simulink model "UAV"  (R2018a)
settings: Solver=VariableStepAuto  StartTime=0.0  StopTime=10.0  RelTol=1e-3
values from neighbouring files (symbols this model uses):
  A = [0 0 1 0 0 0 0.0009 0 0 ... (first row only)    [model.m]    (also in model_disturbance.m)
  B = [0 0 0 ... (first row only)    [model.m]    (also in model_disturbance.m)
  C = [1 0 0 0 0 0 0 0 0 ... (first row only)    [model.m]    (also in model_disturbance.m)
  D = zeros(6,3)    [model.m]    (also in model_disturbance.m = zeros(6,6))
  M = A-B*K-l*C    [model.m]    (also in model_disturbance.m)
undefined symbols (not defined in the file or in its folder): K, l
settings Model: Creator=HP  LastModifiedBy=HP

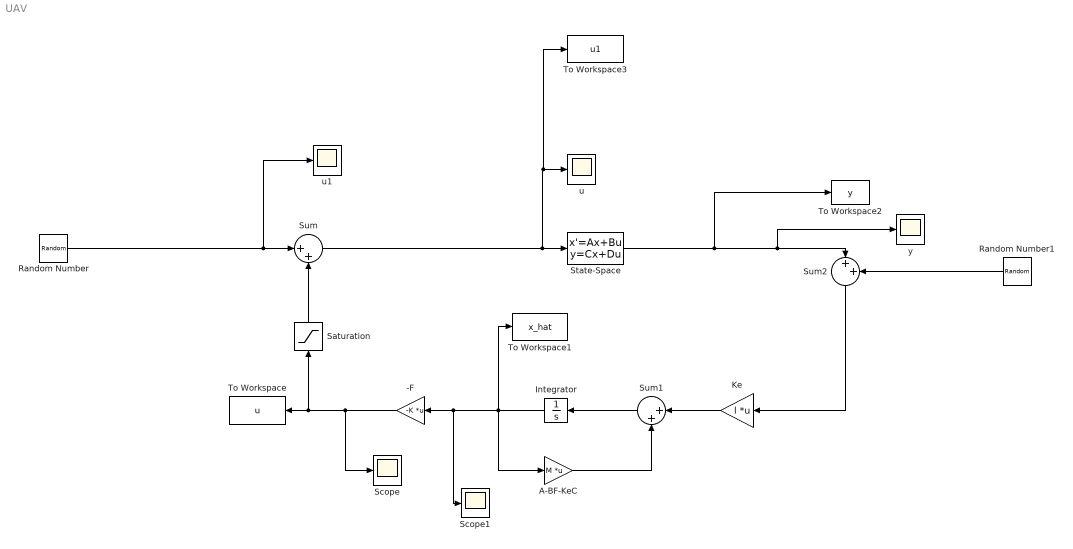
== system UAV ==
  " -F" : Gain  Gain=-K  Multiplication=Matrix(K*u) (u vector)
  A-BF-KeC : Gain  Gain=M  Multiplication=Matrix(K*u) (u vector)
  Integrator : Integrator  InitialCondition=[0 0 0 0 0 0 0 0 0]
  Ke : Gain  Gain=l  Multiplication=Matrix(K*u)
  Random Number : RandomNumber  Variance=0.01  SampleTime=0.1
  Random Number1 : RandomNumber  Variance=0.01  SampleTime=0.1
  Saturation : Saturate
  Scope : Scope
  Scope1 : Scope
  State-Space : StateSpace  A=A  B=B  C=C  D=D  InitialCondition=[0 -0.1 0 0 0 0 0 0 0.1]  ContinuousStateAttributes='plant'
  Sum : Sum  Inputs=|++
  Sum1 : Sum  Inputs=|++
  Sum2 : Sum  Inputs=|++
  To Workspace : ToWorkspace  VariableName=u  SampleTime=-1
  To Workspace1 : ToWorkspace  VariableName=x_hat  SampleTime=-1
  To Workspace2 : ToWorkspace  VariableName=y  SampleTime=-1
  To Workspace3 : ToWorkspace  VariableName=u1  SampleTime=-1
  u : Scope
  u1 : Scope
  y : Scope
  wires:
  Sum1/1 -> Integrator/1
  Sum2/1 -> Ke/1
  A-BF-KeC/1 -> Sum1/2
  Ke/1 -> Sum1/1
  Random Number1/1 -> Sum2/2
  State-Space/1 -> To Workspace2/1, y/1, Sum2/1
  Integrator/1 -> Scope1/1, " -F"/1, A-BF-KeC/1, To Workspace1/1
  " -F"/1 -> Scope/1, To Workspace/1, Saturation/1
  Saturation/1 -> Sum/2
  Random Number/1 -> u1/1, Sum/1
  Sum/1 -> To Workspace3/1, u/1, State-Space/1
